simulink model "weather"  (R2020a)
settings: Solver=FixedStepAuto  StartTime=0.0  StopTime=24*3600  FixedStep=0.01  RelTol=1e-3
PostLoadFcn:
  | if any(exist('dsrtsu_mdlpostloadfcn', 'file') ~= 0), dsrtsu_mdlpostloadfcn('Execute', bdroot); end
InitFcn:
  | , if any(exist('rtifpga_mdlclblib', 'file') ~= 0), rtifpga_mdlclblib('Init', bdroot); end,
  | , if any(exist('dsmpb_private', 'file') ~= 0), dsmpb_private('dsmpb_mdlclblib', 'Init', bdroot); end,
undefined symbols (not defined in the file): dspaceexample_d_dy975jfgkaM
libraries: dsmpblib x2
PreSaveFcn:
  | , if any(exist('dsmpb_private', 'file') ~= 0), dsmpb_private('dsmpb_mdlclblib', 'PreSave', bdroot); end,
CloseFcn:
  | , if any(exist('dsmpb_private', 'file') ~= 0), dsmpb_private('dsmpb_mdlclblib', 'Close', bdroot); end,
settings Model: RTICANMMDATA=struct('GeneralSetupData',struct('modelroot','D:\github\dspace-modelica-example\simulink\weather','generalsettings',struct('filesettings',struct('destfolder',struct('Name','RTICANMM_FILES','Check',1),'buildfolder',struct('Name','.','Check',1),'AbsDestfolder',struct('Name','D:\github\dspace-modelica-example\simulink\weather\RTICANMM_FILES'),'AbsBuildfolder',struct('Name','D:\github\dspace-modelica-example\simulink\weather'))),'options',struct('addpaths',1,'rmpaths',1,'addtrcexclusion',true,'cannavigator',struct('checkmonitoring',0),'show_usrtrc',0,'use_usrtrc',0),'advanced',struct('options',ones(1,100)),'MPSetup',{{}},'RTI',struct('Type','DSRT','Ver','4.3','Date','02-May-2020'),'modelname','weather','block','weather'))  DSRTSU_INTERNAL_RTIFPGA=160  DSMPB_ID_DATA={'85',struct('BlockId','8aff49f3-4eba-4c15-9922-fed59f50903e','SignalIds',{{'f6b20e55-e057-4f6a-a15f-3630c0d4ec6b'}}),'87',struct('BlockId','ac63306b-5b1c-429a-b6fb-42eb2a0b553d','SignalIds',{{'3f132607-5246-475e-85d9-59e57f9eca37'}})}  Creator=yangyang.fu  LastModifiedBy=yangyang.fu
settings OptimizationCC: BlockReduction=off  ConditionallyExecuteInputs=off  OptimizeBlockIOStorage=off  BufferReuse=off
settings DebuggingCC: TasksWithSamePriorityMsg=none
settings HardwareCC: ProdBitPerPointer=32  ProdBitPerSizeT=32  ProdBitPerPtrDiffT=32  ProdLargestAtomicInteger=Integer  ProdWordSize=32  ProdLongLongMode=on  ProdHWDeviceType=Custom Processor->Custom
settings ModelReferenceCC: EnableParallelModelReferenceBuilds=on
settings SFSimCC: MATLABDynamicMemAlloc=off
settings RTWCC: Description=dSPACE Run-Time Target (for VEOS on Windows and ConfigurationDesk)  SystemTargetFile=dsrt.tlc  GenCodeOnly=on  MakeCommand=make_dsrt  TemplateMakefile=dsrt_default_tmf  RTWVerbose=off
settings STFCustomTargetCC: TargetLangStandard=C99 (ISO)  ParMdlRefBuildCompliant=on  SystemTargetFile=dsrt.tlc
settings GRTTargetCC: CompOptLevelCompliant=off  ConcurrentExecutionCompliant=off  CombineOutputUpdateFcns=off  MatFileLogging=off  CPPClassGenCompliant=off  UseToolchainInfoCompliant=off

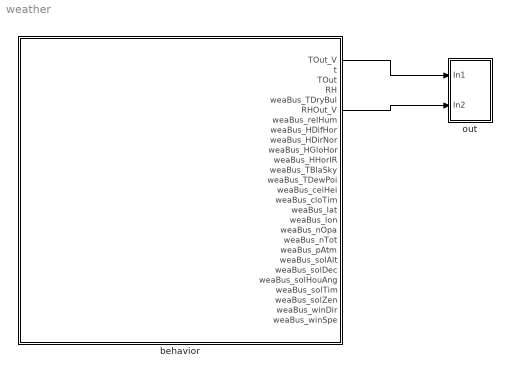
== system weather ==
  behavior : Subsystem
  out : Subsystem
  wires:
  behavior/1(TOut_V) -> out/1(In1)
  behavior/6(RHOut_V) -> out/2(In2)

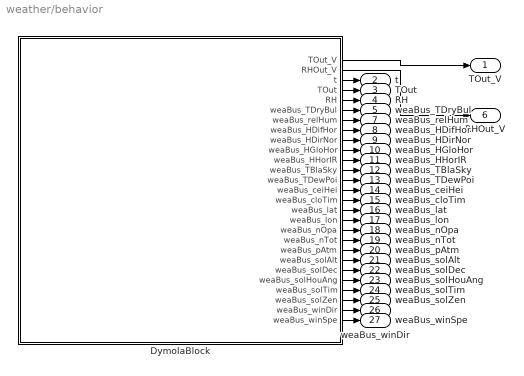
== system weather/behavior ==
  DymolaBlock : Subsystem  Tag=25-Nov-2021 17:00:10#975  LoadFcn=if exist('newDymolaGui') newDymolaGui('weather/behavior/DymolaBlock','PostLoadNew'); else error('Dymola not installed. Must install at least the file newDymolaGui.p'); end;
      mask help:
      | Dymola block.
      | A dymola block allows acausal physical modeling.
      | See Dymola manual for usage.
      settings: CopyFcn=newDymolaGui('25-Nov-2021 17:00:10#975','Copy');  DeleteFcn=if exist('newDymolaGui') newDymolaGui('weather/behavior/DymolaBlock','Delete'); end;  NameChangeFcn=newDymolaGui('25-Nov-2021 17:00:10#975','Copy');  OpenFcn=newDymolaGui('weather/behavior/DymolaBlock','Init');
      mask Display: image(reshape([1;1;1;1;1;1;1;1;1;1;1;1;1;1;1;1;1;1;1;1;1;1;0;0;0;0;0;0;0;0;0;0;1;1;1;1;1;1;1;1;0;1;1;1;1;1;1;1;1;0;1;1;1;1;1;0;0;0;0;0;0;0;1;1;0;0;0;0;0;0;0;1;1;0;0;0;0;0;0;0;1;1;0;0;0;0;0;0;0;1;1;0;0;0;0;0;0;0;1;1;0;0;0;0;0;0;0;1;1;0;0;0;0;0;0;0;1;1;0;0;0;0;0;0;0;1;1;0;0;0;0;0;0;0;1;1;0;0;0;0;0;0;0;1;1;0;0;0;0;0;0;0;1;1;0;0;0;0;0;0;0;1;1;0;0;0;0;0;0;0;1;1;0;0;0;0;0;0;0;1;1;0;0;0;0;0;0;0;1;1;0;0;0;0;0;0;0;1;1;0;0;0;0;0;0;0;1;1;0;0;0;0;0;0;0;1;1;0;0;0;0;0;0;0;1;1;0;0;0;0;0;0;0;1;1;0;0;0;0;0;0;0;1;1;0;0;0;0;0;0;0;1;1;0;0;0;0;0;0;0;1;1;0;0;0;0;0;0;0;1;1;1;1;1;0;1;1;1;1;1;1;1;1;0;1;1;1;1;1;1;1;1;0;0;0;0;0;0;0;0;0;0;1;1;1;1;1;1;1;1;1;1;1;1;1;1;1;1;1;1;1;1;1;1;1;1;1;1;1;1;1;1;1;1;1;1;1;1;1;1;1;1;1;1;1;1;0;0;0;0;0;0;0;0;0;0;1;1;1;1;1;1;1;1;0;1;1;1;1;1;1;1;1;0;1;1;1;1;1;0;0;0;0;0;0;0;1;1;0;0;0;0;0;0;0;1;1;0;0;0;0;0;0;0;1;1;0;0;0;0;0;0;0;1;1;0;0;0;0;0;0;0;1;1;0;0;0;0;0;0;0;1;1;0;0;0;0;0;0;0;1;1;0;0;0;0;0;0;0;1;1;0;0;0;0;0;0;0;1;1;0;0;0;0;0;0;0;1;1;0;0;0;0;0;0;0;1;1;0;0;0;0;0;0;0;1;1;0;0;0;0;0;0;0;1;1;0;0;0;0;0;0;0;1;1;0;0;0;0;0;0;0;1;1;0;0;0;0;0;0;0;1;1;0;0;0;0;0;0;0;1;1;0;0;0;0;0;0;0;1;1;0;0;0;0;0;0;0;1;1;0;0;0;0;0;0;0;1;1;0;0;0;0;0;0;0;1;1;0;0;0;0;0;0;0;1;1;0;0;0;0;0;0;0;1;1;0;0;0;0;0;0;0;1;1;1;1;1;0;1;1;1;1;1;1;1;1;0;1;1;1;1;1;1;1;1;0;0;0;0;0;0;0;0;0;0;1;1;1;1;1;1;1;1;1;1;1;1;1;1;1;1;1;1;1;1;1;1;1;1;1;1;1;1;1;1;1;1;1;1;1;1;1;1;1;1;1;1;1;1;0;0;0;0;0;0;0;0;0;0;1;1;1;1;1;1;1;1;0;1;1;1;1;1;1;1;1;0;1;1;1;1;1;0;0;0;0;0;0;0;1;1;0;0;0;0;0;0;0;1;1;0;1;1;1;1;1;0;1;1;0;1;1;1;1;1;0;1;1;0;1;1;1;1;1;0;1;1;0;1;1;1;1;1;0;1;1;0;1;1;1;1;1;0;1;1;0;1;1;1;1;1;0;1;1;0;1;1;1;1;1;0;1;1;0;1;1;1;1;1;0;1;1;0;1;1;1;1;1;0;1;1;0;1;1;1;1;1;0;1;1;0;1;1;1;1;1;0;1;1;0;1;1;1;1;1;0;1;1;0;1;1;1;1;1;0;1;1;0;1;1;1;1;1;0;1;1;0;1;1;1;1;1;0;1;1;0;1;1;1;1;1;0;1;1;0;1;1;1;1;1;0;1;1;0;1;1;1;1;1;0;1;1;0;1;1;1;1;1;0;1;1;0;1;1;1;1;1;0;1;1;0;0;0;0;0;0;0;1;1;0;0;0;0;0;0;0;1;1;1;1;1;0;1;1;1;1;1;1;1;1;0;1;1;1;1;1;1;1;1;0;0;0;0;0;0;0;0;0;0;1;1;1;1;1;1;1;1;1;1;1;1;1;1;1;1;1;1;1;1;1;1],18,18,3),[.2,.2,.6,.6])
  TOut_V : Outport
  t : Outport  Port=2
  TOut : Outport  Port=3
  RH : Outport  Port=4
  weaBus_TDryBul : Outport  Port=5
  RHOut_V : Outport  Port=6
  weaBus_relHum : Outport  Port=7
  weaBus_HDifHor : Outport  Port=8
  weaBus_HDirNor : Outport  Port=9
  weaBus_HGloHor : Outport  Port=10
  weaBus_HHorIR : Outport  Port=11
  weaBus_TBlaSky : Outport  Port=12
  weaBus_TDewPoi : Outport  Port=13
  weaBus_ceiHei : Outport  Port=14
  weaBus_cloTim : Outport  Port=15
  weaBus_lat : Outport  Port=16
  weaBus_lon : Outport  Port=17
  weaBus_nOpa : Outport  Port=18
  weaBus_nTot : Outport  Port=19
  weaBus_pAtm : Outport  Port=20
  weaBus_solAlt : Outport  Port=21
  weaBus_solDec : Outport  Port=22
  weaBus_solHouAng : Outport  Port=23
  weaBus_solTim : Outport  Port=24
  weaBus_solZen : Outport  Port=25
  weaBus_winDir : Outport  Port=26
  weaBus_winSpe : Outport  Port=27
  wires:
  DymolaBlock/6(weaBus_TDryBul) -> weaBus_TDryBul/1
  DymolaBlock/2(RHOut_V) -> RHOut_V/1
  DymolaBlock/3(t) -> t/1
  DymolaBlock/9(weaBus_HDirNor) -> weaBus_HDirNor/1
  DymolaBlock/4(TOut) -> TOut/1
  DymolaBlock/1(TOut_V) -> TOut_V/1
  DymolaBlock/5(RH) -> RH/1
  DymolaBlock/23(weaBus_solHouAng) -> weaBus_solHouAng/1
  DymolaBlock/17(weaBus_lon) -> weaBus_lon/1
  DymolaBlock/22(weaBus_solDec) -> weaBus_solDec/1
  DymolaBlock/10(weaBus_HGloHor) -> weaBus_HGloHor/1
  DymolaBlock/27(weaBus_winSpe) -> weaBus_winSpe/1
  DymolaBlock/8(weaBus_HDifHor) -> weaBus_HDifHor/1
  DymolaBlock/7(weaBus_relHum) -> weaBus_relHum/1
  DymolaBlock/13(weaBus_TDewPoi) -> weaBus_TDewPoi/1
  DymolaBlock/19(weaBus_nTot) -> weaBus_nTot/1
  DymolaBlock/14(weaBus_ceiHei) -> weaBus_ceiHei/1
  DymolaBlock/12(weaBus_TBlaSky) -> weaBus_TBlaSky/1
  DymolaBlock/11(weaBus_HHorIR) -> weaBus_HHorIR/1
  DymolaBlock/16(weaBus_lat) -> weaBus_lat/1
  DymolaBlock/20(weaBus_pAtm) -> weaBus_pAtm/1
  DymolaBlock/15(weaBus_cloTim) -> weaBus_cloTim/1
  DymolaBlock/21(weaBus_solAlt) -> weaBus_solAlt/1
  DymolaBlock/18(weaBus_nOpa) -> weaBus_nOpa/1
  DymolaBlock/25(weaBus_solZen) -> weaBus_solZen/1
  DymolaBlock/24(weaBus_solTim) -> weaBus_solTim/1
  DymolaBlock/26(weaBus_winDir) -> weaBus_winDir/1

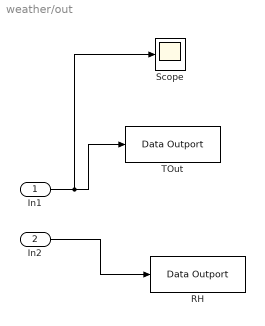
== system weather/out ==
  In1 : Inport
  In2 : Inport  Port=2
  RH : dsmpblib/Data Outport  Priority=-10000
      settings: SourceProductName=dSPACE Model Interface Blockset
  Scope : Scope
  TOut : dsmpblib/Data Outport  Priority=-10000
      settings: SourceProductName=dSPACE Model Interface Blockset
  wires:
  In1/1 -> Scope/1, TOut/1
  In2/1 -> RH/1

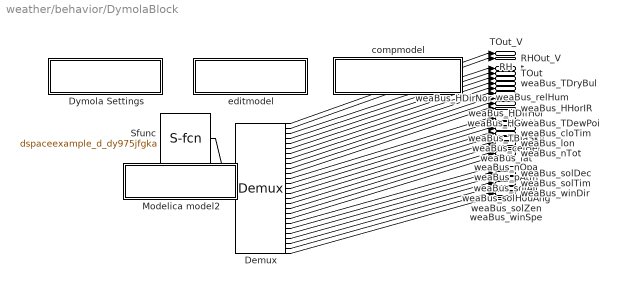
== system weather/behavior/DymolaBlock ==
  Demux : Demux  Outputs=[1;1;1;1;1;1;1;1;1;1;1;1;1;1;1;1;1;1;1;1;1;1;1;1;1;1;1]
  Dymola Settings : Subsystem  mask{ModelName=dSpaceExample.Debug.OA, MoFileName=D:/github/dspace-modelica-example/dSpaceExample/Debug/OA.mo, dSpace=, BusConnector=[], ResultFile=[], ResultFileOnline=[], ResultDt=[], Libs=:, bigobj=[], ImportFolder=[], guimode=[], ModelName2=[], forRuntime=[], MEXLoad=[], omitDescription=[], ResultName=dspaceexample_d_dy975jfgka}
      mask prompts: ModelName "Name of Dymola model"; MoFileName "File Name (including .mo)"; ResultFile "Create Result"; ResultFileOnline "Load result"; ResultDt "Result min dt"; Libs "Used Libraries"; bigobj "Compiler flag /bigobj"; ImportFolder "Import folder"; guimode "GUI mode flag"; ModelName2 "Model name for import mode"; forRuntime "Runtime export"; MEXLoad "Compiled S-function"; omitDescription "Omit description strings"; ResultName "Name of result file"
      mask Display: disp('Dymola Settings');
  Modelica model2 : Subsystem
      mask Display: disp('Change parameters');
  Sfunc : S-Function  Tag=975jfgka  FunctionName=dspaceexample_d_dy975jfgka  Parameters=[dspaceexample_d_dy975jfgkaM.pV],[dspaceexample_d_dy975jfgkaM.x0V]  PortCounts=[0;1]  SFunctionDeploymentMode=off  EnableBusSupport=off
      mask Display: image(imread('Dymola.bmp'))
  compmodel : Subsystem
      settings: OpenFcn=compileModelica('weather/behavior/DymolaBlock');
      mask Display: disp('Compile Modelica model');
  editmodel : Subsystem
      settings: OpenFcn=editModelica('weather/behavior/DymolaBlock');
      mask Display: disp('Edit Modelica model');
  TOut_V : Outport
  RHOut_V : Outport  Port=2
  t : Outport  Port=3
  TOut : Outport  Port=4
  RH : Outport  Port=5
  weaBus_TDryBul : Outport  Port=6
  weaBus_relHum : Outport  Port=7
  weaBus_HDifHor : Outport  Port=8
  weaBus_HDirNor : Outport  Port=9
  weaBus_HGloHor : Outport  Port=10
  weaBus_HHorIR : Outport  Port=11
  weaBus_TBlaSky : Outport  Port=12
  weaBus_TDewPoi : Outport  Port=13
  weaBus_ceiHei : Outport  Port=14
  weaBus_cloTim : Outport  Port=15
  weaBus_lat : Outport  Port=16
  weaBus_lon : Outport  Port=17
  weaBus_nOpa : Outport  Port=18
  weaBus_nTot : Outport  Port=19
  weaBus_pAtm : Outport  Port=20
  weaBus_solAlt : Outport  Port=21
  weaBus_solDec : Outport  Port=22
  weaBus_solHouAng : Outport  Port=23
  weaBus_solTim : Outport  Port=24
  weaBus_solZen : Outport  Port=25
  weaBus_winDir : Outport  Port=26
  weaBus_winSpe : Outport  Port=27
  wires:
  Sfunc/1 -> Demux/1
  Demux/1 -> TOut_V/1
  Demux/2 -> RHOut_V/1
  Demux/3 -> t/1
  Demux/4 -> TOut/1
  Demux/5 -> RH/1
  Demux/6 -> weaBus_TDryBul/1
  Demux/7 -> weaBus_relHum/1
  Demux/8 -> weaBus_HDifHor/1
  Demux/9 -> weaBus_HDirNor/1
  Demux/10 -> weaBus_HGloHor/1
  Demux/11 -> weaBus_HHorIR/1
  Demux/12 -> weaBus_TBlaSky/1
  Demux/13 -> weaBus_TDewPoi/1
  Demux/14 -> weaBus_ceiHei/1
  Demux/15 -> weaBus_cloTim/1
  Demux/16 -> weaBus_lat/1
  Demux/17 -> weaBus_lon/1
  Demux/18 -> weaBus_nOpa/1
  Demux/19 -> weaBus_nTot/1
  Demux/20 -> weaBus_pAtm/1
  Demux/21 -> weaBus_solAlt/1
  Demux/22 -> weaBus_solDec/1
  Demux/23 -> weaBus_solHouAng/1
  Demux/24 -> weaBus_solTim/1
  Demux/25 -> weaBus_solZen/1
  Demux/26 -> weaBus_winDir/1
  Demux/27 -> weaBus_winSpe/1

== system weather/behavior/DymolaBlock/Dymola Settings ==

== system weather/behavior/DymolaBlock/Modelica model2 ==

== system weather/behavior/DymolaBlock/compmodel ==

== system weather/behavior/DymolaBlock/editmodel ==
